simulink model "Calibration_Test_Tx1"  (R2019a)
settings: Solver=FixedStepAuto  StartTime=0.0  StopTime=5  FixedStep=0.001  RelTol=1e-3
libraries: dspnetwork x2
settings Model: Creator=David  LastModifiedBy=David

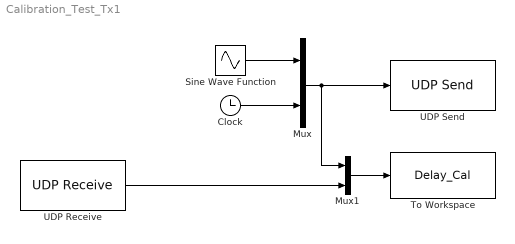
== system Calibration_Test_Tx1 ==
  Clock : Clock
  Mux : Mux  Inputs=2
  Mux1 : Mux  Inputs=2
  Sine Wave Function : Sin  SineType=Sample based  Frequency=3.14  Samples=1000  SampleTime=0.001
  To Workspace : ToWorkspace  VariableName=Delay_Cal  SampleTime=-1
      settings: Save2DSignal=2-D array (concatenate along first dimension)
  UDP Receive : dspnetwork/UDP Receive  localURL='0.0.0.0'  localPort=52050  remoteURL='0.0.0.0'  remotePort=-1  recvBufferSize=16  dims=2  signalDatatype=double  isComplex=off  isVarSize=on  showBlockingTime=off  blockingTime=0  sampletime=0.001  blockPlatform=[]
      settings: SourceProductName=Simulink
  UDP Send : dspnetwork/UDP Send  remoteURL='255.255.255.255'  remotePort=52051  localURL='0.0.0.0'  localPortSource=Automatically determine  localPort=-1  sampletime=-1  blockPlatform=[]  separateLengthPort=0
      settings: SourceProductName=Simulink
  wires:
  Mux/1 -> Mux1/1, UDP Send/1
  Sine Wave Function/1 -> Mux/1
  Clock/1 -> Mux/2
  Mux1/1 -> To Workspace/1
  UDP Receive/1 -> Mux1/2
